simulink subsystem "Var_5"  (R2023a)
settings: Solver=VariableStepAuto  StartTime=0.0  StopTime=10.0  RelTol=1e-3
settings Model: Creator=KozlovM  LastModifiedBy=ПК

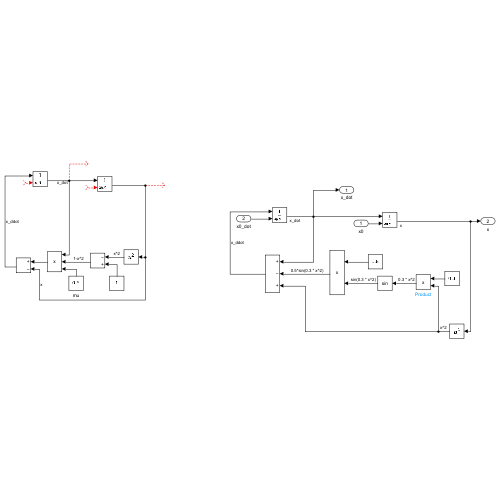
[thumbnail: Simulink's stored preview of the top-level diagram]
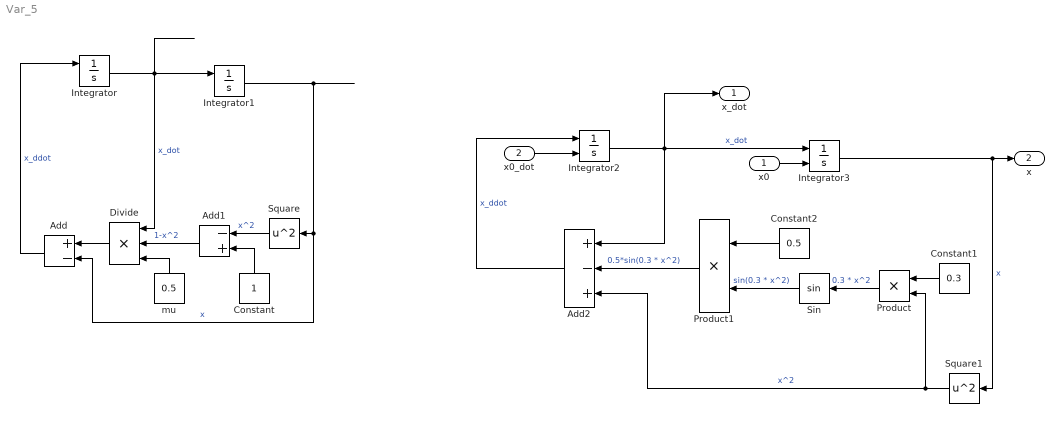
== system Var_5 ==
  x0 : Inport
  x0_dot : Inport  Port=2
  Add : Sum  Inputs=+-
  Add1 : Sum  Inputs=-+
  Add2 : Sum  Inputs=+-+
  Constant : Constant
  Constant1 : Constant  Value=0.3
  Constant2 : Constant  Value=0.5
  Divide : Product  Inputs=***
  Integrator : Integrator  InitialConditionSource=external
  Integrator1 : Integrator  InitialConditionSource=external  InitialCondition=2
  Integrator2 : Integrator  InitialConditionSource=external
  Integrator3 : Integrator  InitialConditionSource=external  InitialCondition=2
  Product : Product
  Product1 : Product
  Sin : Trigonometry
  Square : Math  Operator=square
  Square1 : Math  Operator=square
  mu : Constant  Value=0.5
  x_dot : Outport
  x : Outport  Port=2
  wires:
  Add1/1 -> Divide/2  "1-x^2"
  Constant/1 -> Add1/2
  mu/1 -> Divide/3
  Add/1 -> Integrator/1  "x_ddot"
  Integrator1/1 -> Add/2, Square/1  "x"
  Integrator/1 -> Divide/1, Integrator1/1  "x_dot"
  Square/1 -> Add1/1  "x^2"
  Divide/1 -> Add/1
  ? -> Integrator/2
  ? -> Integrator1/2
  x0_dot/1 -> Integrator2/2
  x0/1 -> Integrator3/2
  Integrator3/1 -> Square1/1, x/1  "x"
  Integrator2/1 -> Add2/1, Integrator3/1, x_dot/1  "x_dot"
  Add2/1 -> Integrator2/1  "x_ddot"
  Square1/1 -> Add2/3, Product/2  "x^2"
  Product/1 -> Sin/1  "0.3 * x^2"
  Constant1/1 -> Product/1
  Sin/1 -> Product1/2  "sin(0.3 * x^2)"
  Constant2/1 -> Product1/1
  Product1/1 -> Add2/2  "0.5*sin(0.3 * x^2)"
